simulink model "regressaround"  (Simulink 7.8)
settings: Solver=ode45  StartTime=0.0  StopTime=10.0  RelTol=1e-3
libraries: StimuliLib x2
settings Model: Creator=Leo  LastModifiedBy=Leo

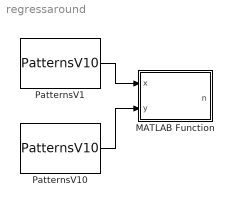
== system regressaround ==
  MATLAB Function : MATLAB Function  TreatAsAtomicUnit=on
  PatternsV1 : StimuliLib/PatternsV10  patternSelection=Hill
  PatternsV10 : StimuliLib/PatternsV10  patternSelection=Hill
  wires:
  PatternsV1/1 -> MATLAB Function/1(x)
  PatternsV10/1 -> MATLAB Function/2(y)

== matlab function MATLAB Function ==
  data: x input double; y input double; n output double
function n = fcn(x,y)
%#codegen
coder.extrinsic('plot');
plot(x,y);
n = 0;
